simulink model "main"  (R2022b)
settings: Solver=FixedStepDiscrete  StartTime=0.0  StopTime=10.0  FixedStep=0.005  RelTol=1e-3
settings Model: ExtModeTrigDuration=2  Creator=F64236C  LastModifiedBy=F64236C
settings OptimizationCC: EnhancedBackFolding=on  PassReuseOutputArgsAs=Individual arguments  ZeroExternalMemoryAtStartup=off  ZeroInternalMemoryAtStartup=off  MaxStackSize=64  OptimizeBlockOrder=speed  DifferentSizesBufferReuse=on  OptimizationCustomize=off  EfficientTunableParamExpr=on
settings DebuggingCC: ParameterTunabilityLossMsg=error
settings HardwareCC: ProdBitPerPointer=32  ProdBitPerSizeT=32  ProdBitPerPtrDiffT=32  ProdLargestAtomicInteger=Long  ProdLargestAtomicFloat=Double  ProdWordSize=32  ProdHWDeviceType=ARM Compatible->ARM Cortex
settings SFSimCC: MATLABDynamicMemAlloc=off
settings RTWCC: Description=Embedded Coder  SystemTargetFile=ert.tlc  HardwareBoard=ESP32-WROOM(Arduino Compatible)  TLCOptions="-aInlineSetEventsForThisBaseRateFcn=TLC_FALSE -aSuppressMultiTaskScheduler=TLC_FALSE  -aRateBasedStepFcn=0"  TemplateMakefile=ert_default_tmf  Toolchain=ESP32  BuildConfiguration=Faster Runs
settings CodeAppCC: ForceParamTrailComments=on  IgnoreCustomStorageClasses=off  OperatorAnnotations=on  SimulinkDataObjDesc=on  SFDataObjDesc=on  InsertBlockDesc=on
settings ERTTargetCC: SupportContinuousTime=on  SupportVariableSizeSignals=on  ExtModeTransport=3  ExtModeStaticAlloc=on  ExtModeAutomaticAllocSize=off  ExtModeStaticAllocSize=65536  ExtModeMexFile=ext_xcp  ExtModeIntrfLevel=Level2 - Open

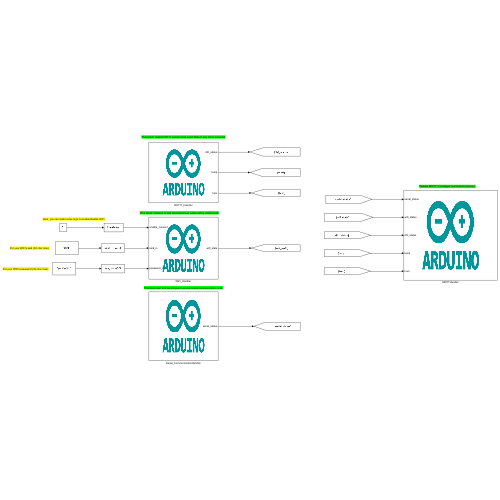
[thumbnail: Simulink's stored preview of the top-level diagram]
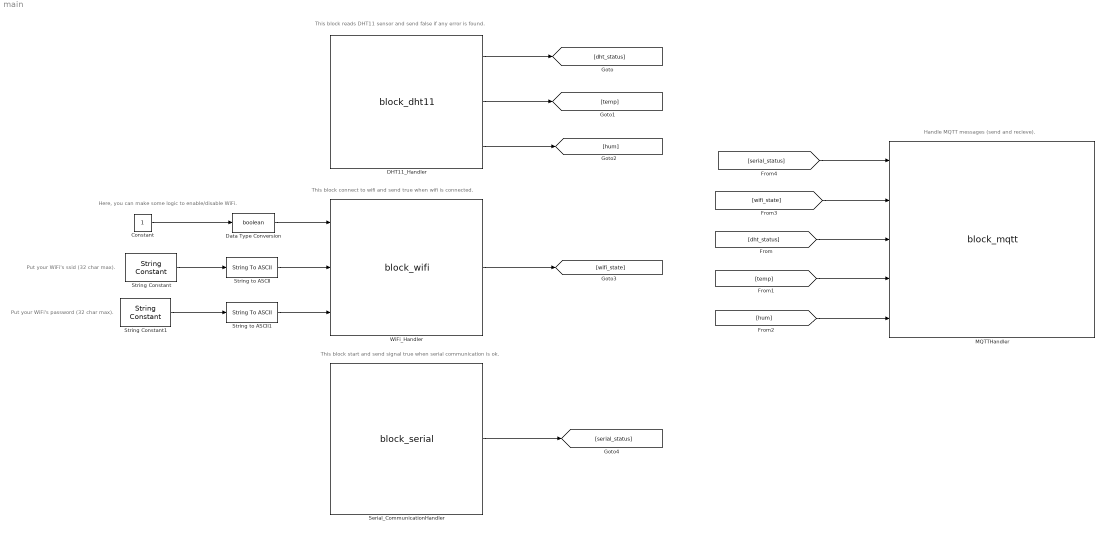
== system main ==
  note: This block connect to wifi and send true when wifi is connected.
  note: This block start and send signal true when serial communication is ok.
  note: Put your WiFi's password (32 char max).
  note: Here, you can make some logic to enable/disable WiFi.
  note: Put your WiFi's ssid (32 char max).
  note: This block reads DHT11 sensor and send false if any error is found.
  note: Handle MQTT messages (send and recieve).
  Constant : Constant
  DHT11_Handler : S-Function  FunctionName=block_dht11  SFunctionModules=block_dht11_wrapper.cpp  SFunctionDeploymentMode=off  EnableBusSupport=off  mask(S-Function Builder){}
      mask help: Simulink:masks:SFunctionBuilder_MD
      mask init:
      | val = [[.9  0.75 0.75 1 1 .9 .9 1]',[1 1 0.75 0.75 .9 .9 1 .9]'];try , sys = get_param(gcb,'SfunBuilderFcnName');if isempty(sys), sys = get_param(gcb,'FunctionName'); end,catch, sys = get_param(gcb,'FunctionName'); end
      settings: CopyFcn=set_param(gcbh,'LinkStatus','none')  OpenFcn=sfunctionwizard(gcbh)
      mask Display:
      | image('../imgs/arduino_logo.png');
      | %plot(val(:,1),val(:,2))
      | %disp(sys)
      | port_label('output',1,'dht_status')
      | port_label('output',2,'temp')
      | port_label('output',3,'hum')
  Data Type Conversion : DataTypeConversion  OutDataTypeStr=boolean  SaturateOnIntegerOverflow=off  RndMeth=Floor
  MQTTHandler : S-Function  FunctionName=block_mqtt  SFunctionModules=block_mqtt_wrapper.cpp  SFunctionDeploymentMode=off  EnableBusSupport=off  mask(S-Function Builder){}
      mask help: Simulink:masks:SFunctionBuilder_MD
      mask init: same as main/DHT11_Handler
      settings: CopyFcn=set_param(gcbh,'LinkStatus','none')  OpenFcn=sfunctionwizard(gcbh)
      mask Display:
      | image('../imgs/arduino_logo.png');
      | 
      | port_label('input',1,'serial_status')
      | port_label('input',2,'wifi_status')
      | port_label('input',3,'dht_status')
      | port_label('input',4,'temp')
      | port_label('input',5,'hum')
  Serial_CommunicationHandler : S-Function  FunctionName=block_serial  SFunctionModules=block_serial_wrapper.cpp  SFunctionDeploymentMode=off  EnableBusSupport=off  mask(S-Function Builder){}
      mask help: Simulink:masks:SFunctionBuilder_MD
      mask init: same as main/DHT11_Handler
      settings: CopyFcn=set_param(gcbh,'LinkStatus','none')  OpenFcn=sfunctionwizard(gcbh)
      mask Display:
      | image('../imgs/arduino_logo.png');
      | %plot(val(:,1),val(:,2))
      | %disp(sys)
      | port_label('output',1,'serial_status')
  String Constant : StringConstant  String="\"ssid\""
  String Constant1 : StringConstant  String="\"password\""
  String to ASCII : StringToASCII  OutputVectorSize=32
  String to ASCII1 : StringToASCII  OutputVectorSize=32
  WiFi_Handler : S-Function  FunctionName=block_wifi  SFunctionModules=block_wifi_wrapper.cpp  SFunctionDeploymentMode=off  EnableBusSupport=off  mask(S-Function Builder){}
      mask help: Simulink:masks:SFunctionBuilder_MD
      mask init: same as main/DHT11_Handler
      settings: CopyFcn=set_param(gcbh,'LinkStatus','none')  OpenFcn=sfunctionwizard(gcbh)
      mask Display:
      | image('../imgs/arduino_logo.png');
      | 
      | port_label('input',1,'enable_connect')
      | port_label('input',2,'ssid_in')
      | port_label('input',3,'password_in')
      | port_label('output',1,'wifi_state')
  wires:
  String to ASCII1/1 -> WiFi_Handler/3
  String to ASCII/1 -> WiFi_Handler/2
  String Constant/1 -> String to ASCII/1
  Data Type Conversion/1 -> WiFi_Handler/1
  String Constant1/1 -> String to ASCII1/1
  Constant/1 -> Data Type Conversion/1
  DHT11_Handler/1 -> [dht_status]
  [dht_status] -> MQTTHandler/3
  DHT11_Handler/2 -> [temp]
  [temp] -> MQTTHandler/4
  DHT11_Handler/3 -> [hum]
  [hum] -> MQTTHandler/5
  WiFi_Handler/1 -> [wifi_state]
  [wifi_state] -> MQTTHandler/2
  Serial_CommunicationHandler/1 -> [serial_status]
  [serial_status] -> MQTTHandler/1
